simulink library "Ampere_Library"  (R2022b)
settings: Solver=FixedStepDiscrete  StartTime=0  StopTime=10.0  RelTol=1e-3  EnableMultiTasking=on
undefined symbols (not defined in the file or in its folder): A_INST_double, Dem_EventStatusType, ECU_AMBIENT_TEMPERATURE, SET_ECU_AMBIENT_TEMPERATURE, SlDemoSign, Std_ReturnType
libraries: simulink x13
(part 6 of 10)

== system Ampere_Library/Basic_Software_Operation/HW_IO/A_HWDiag ==
  note: Block with high width as the function name length depends of the name in the mask.
  note: Refer Mask Description of this Library block for detailed information.
  note: Name and data type updated through mask callback
  PhysicalSampling : FunctionCaller  FunctionPrototype=[ECU_AMBIENT_TEMPERATURE_dg,RTE_Error] = GET_DIAG_AMBIENT_TEMPERATURE()  InputArgumentSpecifications=<Enter example>  OutputArgumentSpecifications=A_INST_double(1),Std_ReturnType(1)
  ECU_AMBIENT_TEMPERATURE_dg : Outport  OutDataTypeStr=double
      settings: AttributesFormatString=DT = %<OutDataTypeStr>
  RTE_Error : Outport  Port=2  OutDataTypeStr=Enum: Std_ReturnType
      settings: AttributesFormatString=DT = %<OutDataTypeStr>
  wires:
  PhysicalSampling/1 -> ECU_AMBIENT_TEMPERATURE_dg/1
  PhysicalSampling/2 -> RTE_Error/1

== system Ampere_Library/Basic_Software_Operation/HW_IO/A_HWInput ==
  note: Block with high width as the function name length depends of the name in the mask.
  note: Name and data type updated through mask callback
  note: Refer Mask Description of this Library block for detailed information.
  PhysicalSampling : FunctionCaller  FunctionPrototype=[ECU_AMBIENT_TEMPERATURE,RTE_Error] = GET_ECU_AMBIENT_TEMPERATURE()  InputArgumentSpecifications=<Enter example>  OutputArgumentSpecifications=A_INST_double(1),Std_ReturnType(1)
  ECU_AMBIENT_TEMPERATURE : Outport  OutDataTypeStr=double
      settings: AttributesFormatString=DT = %<OutDataTypeStr>
  RTE_Error : Outport  Port=2  OutDataTypeStr=Enum: Std_ReturnType
      settings: AttributesFormatString=DT = %<OutDataTypeStr>
  wires:
  PhysicalSampling/2 -> RTE_Error/1
  PhysicalSampling/1 -> ECU_AMBIENT_TEMPERATURE/1

== system Ampere_Library/Basic_Software_Operation/HW_IO/A_HWOutput ==
  note: Name updated through mask callback
  note: Block with high width as the function name length depends of the name in the mask.
  note: Refer Mask Description of this Library block for detailed information.
  ECU_AMBIENT_TEMPERATURE : Inport
  PhysicalSampling : FunctionCaller  FunctionPrototype=SET_ECU_AMBIENT_TEMPERATURE(ECU_AMBIENT_TEMPERATURE)  InputArgumentSpecifications=A_INST_double(1)  OutputArgumentSpecifications=<Enter example>
  wires:
  ECU_AMBIENT_TEMPERATURE/1 -> PhysicalSampling/1

== system Ampere_Library/MBD_Base_Blocks/Simulink/CommonlyUsedBlocks ==
  note: Commonly used blocks
  In : Inport
  Add : Sum  InputSameDT=on  RndMeth=Zero
  Bus_Creator : BusCreator  Inputs=2
  Bus_Selector : BusSelector  OutputSignals=signal1,signal2
  Cons_val : Constant  Value=0
  Data_Type_Conversion : DataTypeConversion  SaturateOnIntegerOverflow=off
  Demux : Demux  Outputs=2
  Logical_Operator : Logic  OutDataTypeStr=boolean
  Mux : Mux  Inputs=2
  Product : Product  RndMeth=Zero
  Relational_Operator : RelationalOperator  Operator=<=  OutDataTypeStr=boolean  RndMeth=Zero
  Saturation : Saturate  RndMeth=Zero
      settings: AttributesFormatString=Max = %<UpperLimit>\nMin = %<LowerLimit>\n
  Subsystem : Subsystem
      settings: CopyFcn=set_param(gcbh,'LinkStatus','none'); set_param(gcbh,'Mask','off'); set_param(gcbh,'MaskType',''); set_param(gcbh,'MaskDescription',''); set_param(gcbh,'OpenFcn',''); set_param(gcbh,'CopyFcn','');  OpenFcn=open_system(gcbh,'force');
  Switch : Switch  Criteria=u2 ~= 0  RndMeth=Zero  SaturateOnIntegerOverflow=off
  Terminator : Terminator
  VectorConcat : Concatenate
  Out : Outport

== system Ampere_Library/MBD_Base_Blocks/Simulink/Discontinuities ==
  note: Discontinuities
  Dead_Zone : DeadZone  SaturateOnIntegerOverflow=off
      settings: AttributesFormatString=|
      | Start = %<LowerValue>
      | End = %<UpperValue>
  RateLimiter : RateLimiter  SampleTimeMode=inherited
      settings: AttributesFormatString=Init = %<InitialCondition>
  Relay : Relay
      settings: AttributesFormatString=|
      | Switch On = %<OnSwitchValue>
      | Switch Off = %<OffSwitchValue>
  Saturation : Saturate  RndMeth=Zero
      settings: AttributesFormatString=Max = %<UpperLimit>\nMin = %<LowerLimit>\n
  Saturation_Dynamic : simulink/Discontinuities/Saturation Dynamic  OutMin=[]  OutMax=[]  OutDataTypeStr=Inherit: Same as second input  OutDataType=fixdt(1, 16)  OutScaling=2^-10  RndMeth=Zero  DoSatur=off

== system Ampere_Library/MBD_Base_Blocks/Simulink/Discrete ==
  note: Discrete
  Delay : Delay  InitialCondition=0
      settings: AttributesFormatString=|
      | Init = %<InitialCondition>
      | Length = %<DelayLength>
  Discrete_State_Space : DiscreteStateSpace  SampleTime=-1
      settings: AttributesFormatString=Init = %<X0>
  TappedDelay : simulink/Discrete/Tapped Delay  vinit=0.0  samptime=-1  NumDelays=4  DelayOrder=Oldest  includeCurrent=off
      settings: AttributesFormatString=|
      | IC = %<vinit>
      | Tapped Order = %<DelayOrder>
  Unit_Delay : UnitDelay  SampleTime=-1  HasFrameUpgradeWarning=on
      settings: AttributesFormatString=Init = %<InitialCondition>

== system Ampere_Library/MBD_Base_Blocks/Simulink/Logic_and_Bit_Operations ==
  note: Logic and Bit Operations
  Bit_Clear : simulink/Logic and Bit Operations/Bit Clear  iBit=0
      settings: AttributesFormatString=ith Bit = %<iBit>
  Bit_Set : simulink/Logic and Bit Operations/Bit Set  iBit=0
      settings: AttributesFormatString=ith Bit = %<iBit>
  Bitwise_Operator : simulink/Logic and Bit Operations/Bitwise Operator  logicop=AND  UseBitMask=on  BitMask=217  BitMaskRealWorld=Stored Integer
      settings: AttributesFormatString=Bit Mask = %<BitMask>\n
  Extract_Bits : simulink/Logic and Bit Operations/Extract Bits  bitsToExtract=Range starting with most significant bit  numBits=8  bitIdxRange=[0 7]  outScalingMode=Treat bit field as an integer
      settings: AttributesFormatString=No of bits = %<numBits>
  Logical_Operator : Logic  OutDataTypeStr=boolean
  Relational_Operator : RelationalOperator  Operator=<=  OutDataTypeStr=boolean  RndMeth=Zero
  Shift_Arithmetic : ArithShift  BitShiftNumber=8

== system Ampere_Library/MBD_Base_Blocks/Simulink/Lookup_Tables ==
  note: Lookup Tables
  Direct_Lookup_Table_n_D : LookupNDDirect  DiagnosticForOutOfRangeInput=None
      settings: AttributesFormatString=Table = %<Table>
  InterpolationUsingPrelookup : Interpolation_n-D  ExtrapMethod=Clip  ValidIndexMayReachLast=on  InternalRulePriority=Speed
      settings: AttributesFormatString=Table = %<Table>
  LookupTableDynamic : simulink/Lookup Tables/Lookup Table Dynamic  LookUpMeth=Interpolation-Use End Values  OutDataType=fixdt('double')  OutScaling=[]  OutputDataTypeScalingMode=Specify via dialog  OutDataTypeStr=double  RndMeth=Zero  DoSatur=off
      settings: AttributesFormatString=DT = %<OutDataTypeStr>
  One_D_Lookup_Table : Lookup_n-D  NumberOfTableDimensions=1  BreakpointsForDimension1=[-5:5]  Table=tanh([-5:5])  ExtrapMethod=Clip  UseLastTableValue=on  InternalRulePriority=Speed  OutDataTypeStr=Inherit: Inherit from 'Table data'  RndMeth=Zero
      settings: AttributesFormatString=|
      | Table = %<Table>
      | X = %<BreakpointsForDimension1>
  Prelookup : PreLookup  BreakpointsData=[10:10:110]  UseLastBreakpoint=on  FractionDataTypeStr=fixdt(1,32,0)
      settings: AttributesFormatString=X = %<BreakpointsData>
  Two_D_Lookup_Table : Lookup_n-D  BreakpointsForDimension1=[1:3]  BreakpointsForDimension2=[1:3]  ExtrapMethod=Clip  UseLastTableValue=on  InternalRulePriority=Speed  OutDataTypeStr=Inherit: Inherit from 'Table data'  RndMeth=Zero
      settings: InputPortMap=u0,u1
      settings: AttributesFormatString=|
      | Table = %<Table>
      | X = %<BreakpointsForDimension1>
      | Y = %<BreakpointsForDimension2>

== system Ampere_Library/MBD_Base_Blocks/Simulink/Math_Operations ==
  note: Math Operations
  Abs : Abs  RndMeth=Zero  SaturateOnIntegerOverflow=off
  Add : Sum  InputSameDT=on  RndMeth=Zero
  Assignment : Assignment  IndexMode=Zero-based  IndexOptions=Index vector (dialog)  Indices=1  OutputSizes=1
      settings: AttributesFormatString=Index Mode = %<IndexMode>\n
  Divide : Product  Inputs=*/  RndMeth=Zero
  MatrixConcatenate : Concatenate  Mode=Multidimensional array  ConcatenateDimension=2
  MinMax : MinMax  InputSameDT=on  RndMeth=Zero
  Permute Dimensions : PermuteDimensions
  Product : Product  RndMeth=Zero
  Product_of_Elements : Product  Inputs=*  RndMeth=Zero
  Reshape : Reshape
  Sign : Signum
  Subtract : Sum  Inputs=+-  InputSameDT=on  RndMeth=Zero
  Sum_of_Elements : Sum  Inputs=+  InputSameDT=on  RndMeth=Zero
  VectorConcatenate : Concatenate

== system Ampere_Library/MBD_Base_Blocks/Simulink/Model_Wide_Utilities ==
  note: Model Wide Utilities
  DocBlock : simulink/Model-Wide Utilities/DocBlock  DocumentType=Text
      content=|
      | Type your documentation here
  ModelInfo : simulink/Model-Wide Utilities/Model Info  Frame=on  DisplayStringWithTags=Model Info  HorizontalTextAlignment=Center  LeftAlignmentValue=0.5

== system Ampere_Library/MBD_Base_Blocks/Simulink/Ports_and_Subsystems ==
  note: Ports & Subsystems
  In1 : Inport
  Enable : EnablePort
      settings: AttributesFormatString=%<StatesWhenEnabling>\n
  Trigger : TriggerPort  VariantControl=Variant  PortDimensions=1
  Atomic_Subsystem : Subsystem  TreatAsAtomicUnit=on
      settings: CopyFcn=set_param(gcbh,'LinkStatus','none'); set_param(gcbh,'Mask','off'); set_param(gcbh,'MaskType',''); set_param(gcbh,'MaskDescription',''); set_param(gcbh,'OpenFcn',''); set_param(gcbh,'CopyFcn','');  OpenFcn=open_system(gcbh,'force');
  CodeReuseSubsystem : Subsystem  TreatAsAtomicUnit=on
      settings: CopyFcn=set_param(gcbh,'LinkStatus','none'); set_param(gcbh,'Mask','off'); set_param(gcbh,'MaskType',''); set_param(gcbh,'MaskDescription',''); set_param(gcbh,'OpenFcn',''); set_param(gcbh,'CopyFcn','');  OpenFcn=open_system(gcbh,'force');  RTWFcnNameOpts=Use subsystem name  RTWFileNameOpts=Use function name
  Enabled_Subsystem : Subsystem  TreatAsAtomicUnit=on
      settings: CopyFcn=set_param(gcbh,'LinkStatus','none'); set_param(gcbh,'Mask','off'); set_param(gcbh,'MaskType',''); set_param(gcbh,'MaskDescription',''); set_param(gcbh,'OpenFcn',''); set_param(gcbh,'CopyFcn','');  OpenFcn=open_system(gcbh,'force');
  Enabled_and_Triggered_Subsystem : Subsystem  TreatAsAtomicUnit=on
      settings: CopyFcn=set_param(gcbh,'LinkStatus','none'); set_param(gcbh,'Mask','off'); set_param(gcbh,'MaskType',''); set_param(gcbh,'MaskDescription',''); set_param(gcbh,'OpenFcn',''); set_param(gcbh,'CopyFcn','');  OpenFcn=open_system(gcbh,'force');
  ForEachSubsystem : Subsystem  TreatAsAtomicUnit=on
      settings: CopyFcn=set_param(gcbh,'LinkStatus','breakWithoutHierarchy'); set_param(gcbh,'Mask','off'); set_param(gcbh,'MaskType',''); set_param(gcbh,'MaskDescription',''); set_param(gcbh,'OpenFcn',''); set_param(gcbh,'CopyFcn','')
  For_Iterator_Subsystem : Subsystem  TreatAsAtomicUnit=on
      settings: CopyFcn=set_param(gcbh,'LinkStatus','none'); set_param(gcbh,'Mask','off'); set_param(gcbh,'MaskType',''); set_param(gcbh,'MaskDescription',''); set_param(gcbh,'OpenFcn',''); set_param(gcbh,'CopyFcn','');  OpenFcn=open_system(gcbh,'force');
  Function_Call_Subsystem : Subsystem  TreatAsAtomicUnit=on
      settings: CopyFcn=set_param(gcbh,'LinkStatus','none'); set_param(gcbh,'Mask','off'); set_param(gcbh,'MaskType',''); set_param(gcbh,'MaskDescription',''); set_param(gcbh,'OpenFcn',''); set_param(gcbh,'CopyFcn','');  OpenFcn=open_system(gcbh,'force');
  If : If
  If_Action_Subsystem : Subsystem  TreatAsAtomicUnit=on
      settings: CopyFcn=set_param(gcbh,'LinkStatus','none'); set_param(gcbh,'Mask','off'); set_param(gcbh,'MaskType',''); set_param(gcbh,'MaskDescription',''); set_param(gcbh,'OpenFcn',''); set_param(gcbh,'CopyFcn','');  OpenFcn=open_system(gcbh,'force');
  Model : ModelReference  SimulationMode=Normal
  Model_Variants : Subsystem  Variant=on
      settings: AttributesFormatString=Active variants=%<ActiveVariant>\n
  Subsystem : Subsystem
      settings: CopyFcn=set_param(gcbh,'LinkStatus','none'); set_param(gcbh,'Mask','off'); set_param(gcbh,'MaskType',''); set_param(gcbh,'MaskDescription',''); set_param(gcbh,'OpenFcn',''); set_param(gcbh,'CopyFcn','');  OpenFcn=open_system(gcbh,'force');
  Switch_Case : SwitchCase
  Switch_Case_Action_Subsystem : Subsystem  TreatAsAtomicUnit=on
      settings: CopyFcn=set_param(gcbh,'LinkStatus','none'); set_param(gcbh,'Mask','off'); set_param(gcbh,'MaskType',''); set_param(gcbh,'MaskDescription',''); set_param(gcbh,'OpenFcn',''); set_param(gcbh,'CopyFcn','');  OpenFcn=open_system(gcbh,'force');
  Triggered_Subsystem : Subsystem  TreatAsAtomicUnit=on
      settings: CopyFcn=set_param(gcbh,'LinkStatus','none'); set_param(gcbh,'Mask','off'); set_param(gcbh,'MaskType',''); set_param(gcbh,'MaskDescription',''); set_param(gcbh,'OpenFcn',''); set_param(gcbh,'CopyFcn','');  OpenFcn=open_system(gcbh,'force');
  Variant_subsystem : Subsystem  Variant=on
      settings: AttributesFormatString=Active variants=%<ActiveVariant>\n  CopyFcn=set_param(gcbh,'LinkStatus','none'); set_param(gcbh,'Mask','off'); set_param(gcbh,'MaskType',''); set_param(gcbh,'MaskDescription',''); set_param(gcbh,'OpenFcn',''); set_param(gcbh,'CopyFcn','');
  While_Iterator_Subsystem : Subsystem  TreatAsAtomicUnit=on
      settings: CopyFcn=set_param(gcbh,'LinkStatus','none'); set_param(gcbh,'Mask','off'); set_param(gcbh,'MaskType',''); set_param(gcbh,'MaskDescription',''); set_param(gcbh,'OpenFcn',''); set_param(gcbh,'CopyFcn','');  OpenFcn=open_system(gcbh,'force');
  Out1 : Outport

== system Ampere_Library/MBD_Base_Blocks/Simulink/Signal_Attributes ==
  note: Signal Attributes
  BustoVector : BusToVector
  DataTypeDuplicate : DataTypeDuplicate
  Data_Type_Conversion : DataTypeConversion  SaturateOnIntegerOverflow=off
  SignalConversion : SignalConversion  OverrideOpt=off

== system Ampere_Library/MBD_Base_Blocks/Simulink/Signal_Routing ==
  note: Signal Routing
  BusAssignment : BusAssignment  AssignedSignals=signal1
  Bus_Creator : BusCreator  Inputs=2
      settings: CopyFcn=set_param(gcbh,'ShowName','off','CopyFcn','')
  Bus_Selector : BusSelector  OutputSignals=signal1,signal2
      settings: CopyFcn=set_param(gcbh,'ShowName','off','CopyFcn','')
  Demux : Demux  Outputs=2
      settings: CopyFcn=set_param(gcbh,'ShowName','off','CopyFcn','')
  From : From
  Goto : Goto
  IndexVector : MultiPortSwitch  DataPortOrder=Zero-based contiguous  Inputs=1  zeroidx=on  RndMeth=Zero  SaturateOnIntegerOverflow=off
  Merge : Merge
      settings: AttributesFormatString=Init = %<InitialOutput>
  Multiport_Switch : MultiPortSwitch  DataPortOrder=Zero-based contiguous  DataPortForDefault=Additional data port  DiagnosticForDefault=None  zeroidx=on  RndMeth=Zero  SaturateOnIntegerOverflow=off
  Mux : Mux  Inputs=2
      settings: CopyFcn=set_param(gcbh,'ShowName','off','CopyFcn','')
  Selector : Selector  IndexMode=Zero-based  IndexOptions=Index vector (port)  Indices=[1 3]  OutputSizes=1
  Switch : Switch  Criteria=u2 ~= 0  RndMeth=Zero  SaturateOnIntegerOverflow=off

== system Ampere_Library/MBD_Base_Blocks/Simulink/Sinks ==
  note: Sinks
  Terminator : Terminator
  Out : Outport

== system Ampere_Library/MBD_Base_Blocks/Simulink/Sources ==
  note: Sources
  In : Inport
  Constant : Constant  Value=0
  EnumeratedConstant : simulink/Sources/Enumerated Constant  OutDataTypeStr=Enum: SlDemoSign  Value=SlDemoSign.Positive  SampleTime=inf
      settings: AttributesFormatString=Enum
  Ground : Ground

== system Ampere_Library/MBD_Base_Blocks/Simulink/User_Defined_Functions ==
  note: User_Defined_Functions
  FunctionCaller : FunctionCaller  FunctionPrototype=y = f(u)  InputArgumentSpecifications=<Enter example>  OutputArgumentSpecifications=<Enter example>
  Initialize_Function : Subsystem  TreatAsAtomicUnit=on
  MATLAB_Function : MATLAB Function  TreatAsAtomicUnit=on
  Simulink_Function : Subsystem  TreatAsAtomicUnit=on
      settings: CopyFcn=set_param(gcbh,'LinkStatus','breakWithoutHierarchy'); set_param(gcbh,'Mask','off'); set_param(gcbh,'MaskType',''); set_param(gcbh,'MaskDescription',''); set_param(gcbh,'OpenFcn',''); set_param(gcbh,'CopyFcn','')

== system Ampere_Library/User_Defined_Libraries/Discontinuities/A_DetectSaturation ==
  note: Refer Mask Description of this Library block for detailed information.
  Upper : Inport
  In : Inport  Port=2
  Lower : Inport  Port=3
  LogicalOperator : Logic  OutDataTypeStr=boolean
  LogicalOperator1 : Logic  Operator=NOT  OutDataTypeStr=boolean
  LogicalOperator2 : Logic  Operator=NOT  OutDataTypeStr=boolean
  Max : MinMax  Function=max  Inputs=2  InputSameDT=on  RndMeth=Zero
      settings: AttributesFormatString=SAT = %<SaturateOnIntegerOverflow>
  Min : MinMax  Inputs=2  InputSameDT=on  RndMeth=Zero
      settings: AttributesFormatString=SAT = %<SaturateOnIntegerOverflow>
  RelationalOperator2 : RelationalOperator  Operator=>  OutDataTypeStr=boolean  RndMeth=Zero
  RelationalOperator3 : RelationalOperator  Operator=<  OutDataTypeStr=boolean  RndMeth=Zero
  RelationalOperator4 : RelationalOperator  Operator=<=  OutDataTypeStr=boolean  RndMeth=Zero
  RelationalOperator5 : RelationalOperator  OutDataTypeStr=boolean  RndMeth=Zero
  SATMAX : Constant  Value=SatMax
  SATMAX1 : Constant  Value=SatMax
  SATMIN : Constant  Value=Satmin
  SATPAS : Constant  Value=SatPas
  Switch{1..4} (4 alike) : Switch  Criteria=u2 ~= 0  RndMeth=Zero  SaturateOnIntegerOverflow=off
  UP_EQ_LOW : Constant  Value=UpEqLow
  Out : Outport
  sat : Outport  Port=2
  wires:
  Lower/1 -> Max/2, [Lower]
  Min/1 -> Out/1, RelationalOperator4/1, RelationalOperator5/1
  [Lower] -> RelationalOperator4/2
  Max/1 -> Min/1
  [Upper] -> RelationalOperator5/2
  LogicalOperator2/1 -> LogicalOperator/1
  Upper/1 -> [Upper], Min/2
  SATPAS/1 -> Switch4/3
  Switch1/1 -> Switch3/3
  [Upper] -> RelationalOperator2/1, RelationalOperator3/1
  RelationalOperator2/1 -> LogicalOperator2/1
  SATMAX1/1 -> Switch3/1
  Switch2/1 -> sat/1
  RelationalOperator4/1 -> Switch4/2
  RelationalOperator3/1 -> LogicalOperator1/1, Switch3/2
  RelationalOperator5/1 -> Switch1/2
  Switch3/1 -> Switch2/3
  SATMAX/1 -> Switch1/1
  [Lower] -> RelationalOperator2/2, RelationalOperator3/2
  In/1 -> Max/1
  LogicalOperator1/1 -> LogicalOperator/2
  LogicalOperator/1 -> Switch2/2
  UP_EQ_LOW/1 -> Switch2/1
  Switch4/1 -> Switch1/3
  SATMIN/1 -> Switch4/1

== system Ampere_Library/User_Defined_Libraries/Discontinuities/A_HiThresHys_HighIncl ==
  note: Refer Mask Description of this Library block for detailed information.
  note: hflg = OFF
  note: hflg = ON
  val : Inport
  thrs : Inport  Port=2
  hysw : Inport  Port=3
  NOT : Logic  Operator=NOT  Inputs=1  OutDataTypeStr=boolean
  RelOperator1 : RelationalOperator  Operator=>  OutDataTypeStr=boolean  RndMeth=Zero
  RelOperator2 : RelationalOperator  Operator=<  OutDataTypeStr=boolean  RndMeth=Zero
  Sum : Sum  InputSameDT=on  RndMeth=Zero
      settings: AttributesFormatString=SAT = %<SaturateOnIntegerOverflow>
  Switch : Switch  Criteria=u2 ~= 0  RndMeth=Zero  SaturateOnIntegerOverflow=off
  Unit_Delay : UnitDelay  InitialCondition=Initial_condition  SampleTime=-1  HasFrameUpgradeWarning=on
      settings: AttributesFormatString=Init = %<InitialCondition>\n
  flag : Outport
  wires:
  NOT/1 -> flag/1, Unit_Delay/1
  Unit_Delay/1 -> Switch/2
  RelOperator2/1 -> Switch/3
  RelOperator1/1 -> Switch/1
  hysw/1 -> Sum/2
  Switch/1 -> NOT/1
  Sum/1 -> RelOperator1/2
  thrs/1 -> RelOperator1/1, RelOperator2/2
  val/1 -> RelOperator2/1, Sum/1

== system Ampere_Library/User_Defined_Libraries/Discontinuities/A_HiThresHys_LowIncl ==
  note: Refer Mask Description of this Library block for detailed information.
  note: hflg = OFF
  note: hflg = ON
  val : Inport
  thrs : Inport  Port=2
  hysw : Inport  Port=3
  NOT : Logic  Operator=NOT  Inputs=1  OutDataTypeStr=boolean
  RelationOperator1 : RelationalOperator  Operator=<=  OutDataTypeStr=boolean  RndMeth=Zero
  RelationalOperator : RelationalOperator  OutDataTypeStr=boolean  RndMeth=Zero
  Sum : Sum  InputSameDT=on  RndMeth=Zero
      settings: AttributesFormatString=SAT = %<SaturateOnIntegerOverflow>
  Switch : Switch  Criteria=u2 ~= 0  RndMeth=Zero  SaturateOnIntegerOverflow=off
  Unit_Delay : UnitDelay  InitialCondition=Initial_condition  SampleTime=-1  HasFrameUpgradeWarning=on
      settings: AttributesFormatString=Init = %<InitialCondition>\n
  flag : Outport
  wires:
  NOT/1 -> flag/1, Unit_Delay/1
  Unit_Delay/1 -> Switch/2
  RelationOperator1/1 -> Switch/3
  RelationalOperator/1 -> Switch/1
  hysw/1 -> Sum/2
  Switch/1 -> NOT/1
  Sum/1 -> RelationalOperator/2
  val/1 -> RelationOperator1/1, Sum/1
  thrs/1 -> RelationalOperator/1, RelationOperator1/2

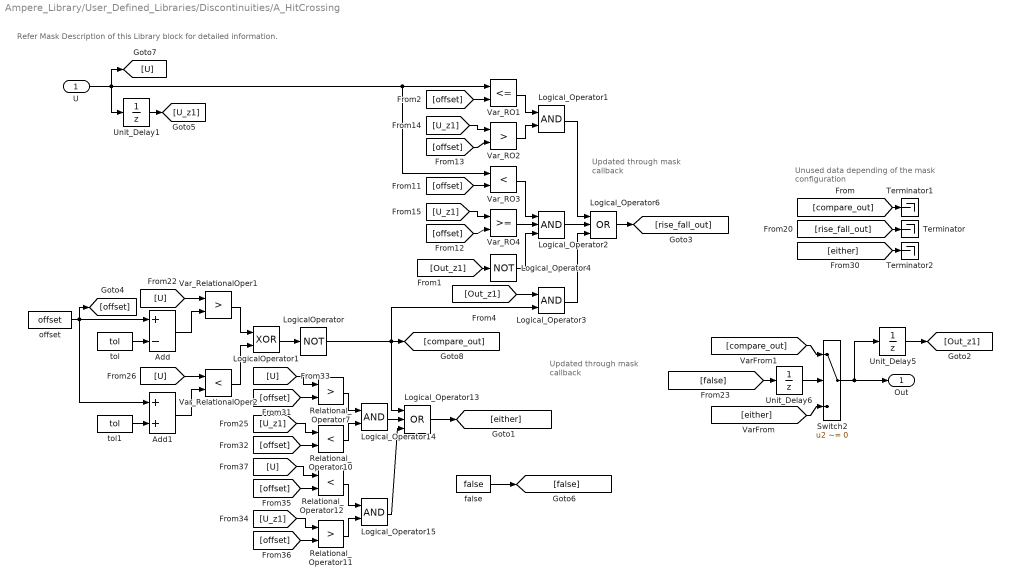
== system Ampere_Library/User_Defined_Libraries/Discontinuities/A_HitCrossing ==
  note: Updated through
      | mask callback
  note: Refer Mask Description of this Library block for detailed information.
  note: Unused data depending
      | of the mask configuration
  note: Updated through
      | mask callback
  U : Inport
  Add : Sum  Inputs=+-  InputSameDT=on  RndMeth=Zero
      settings: AttributesFormatString=SAT = %<SaturateOnIntegerOverflow>
  Add1 : Sum  InputSameDT=on  RndMeth=Zero
      settings: AttributesFormatString=SAT = %<SaturateOnIntegerOverflow>
  LogicalOperator : Logic  Operator=NOT  OutDataTypeStr=boolean
  LogicalOperator1 : Logic  Operator=XOR  OutDataTypeStr=boolean
  Logical_Operator{1,3,14..15} (4 alike) : Logic  OutDataTypeStr=boolean
  Logical_Operator13 : Logic  Operator=OR  Inputs=3  OutDataTypeStr=boolean
  Logical_Operator2 : Logic  Inputs=3  OutDataTypeStr=boolean
  Logical_Operator4 : Logic  Operator=NOT  OutDataTypeStr=boolean
  Logical_Operator6 : Logic  Operator=OR  Inputs=3  OutDataTypeStr=boolean
  Relational_Operator10 : RelationalOperator  Operator=<  OutDataTypeStr=boolean  RndMeth=Zero
  Relational_Operator11 : RelationalOperator  Operator=>  OutDataTypeStr=boolean  RndMeth=Zero
  Relational_Operator12 : RelationalOperator  Operator=<  OutDataTypeStr=boolean  RndMeth=Zero
  Relational_Operator7 : RelationalOperator  Operator=>  OutDataTypeStr=boolean  RndMeth=Zero
  Switch2 : Switch  Criteria=u2 ~= 0  RndMeth=Zero  SaturateOnIntegerOverflow=off
  Terminator : Terminator
  Terminator1 : Terminator
  Terminator2 : Terminator
  Unit_Delay1 : UnitDelay  InitialCondition=INI_VAL  SampleTime=-1  HasFrameUpgradeWarning=on
      settings: AttributesFormatString=Init = %<InitialCondition>
  Unit_Delay5 : UnitDelay  InitialCondition=false  SampleTime=-1  HasFrameUpgradeWarning=on
      settings: AttributesFormatString=Init = %<InitialCondition>
  Unit_Delay6 : UnitDelay  InitialCondition=true  SampleTime=-1  HasFrameUpgradeWarning=on
      settings: AttributesFormatString=Init = %<InitialCondition>
  Var_RO1 : RelationalOperator  Operator=<=  OutDataTypeStr=boolean  RndMeth=Zero
  Var_RO2 : RelationalOperator  Operator=>  OutDataTypeStr=boolean  RndMeth=Zero
  Var_RO3 : RelationalOperator  Operator=<  OutDataTypeStr=boolean  RndMeth=Zero
  Var_RO4 : RelationalOperator  OutDataTypeStr=boolean  RndMeth=Zero
  Var_RelationalOper1 : RelationalOperator  Operator=>  OutDataTypeStr=boolean  RndMeth=Zero
  Var_RelationalOper2 : RelationalOperator  Operator=<  OutDataTypeStr=boolean  RndMeth=Zero
  false : Constant  Value=false
  offset : Constant  Value=offset  OutDataTypeStr=Inherit: Inherit via back propagation
  tol : Constant  Value=tol  OutDataTypeStr=Inherit: Inherit via back propagation
  tol1 : Constant  Value=tol  OutDataTypeStr=Inherit: Inherit via back propagation
  Out : Outport
  wires:
  [offset] -> Relational_Operator7/2
  Var_RO1/1 -> Logical_Operator1/1
  Logical_Operator6/1 -> [rise_fall_out]
  Unit_Delay5/1 -> [Out_z1]
  Var_RelationalOper2/1 -> LogicalOperator1/2
  LogicalOperator1/1 -> LogicalOperator/1
  Var_RO2/1 -> Logical_Operator1/2
  Add1/1 -> Var_RelationalOper2/2
  Unit_Delay1/1 -> [U_z1]
  [false] -> Unit_Delay6/1
  [compare_out] -> Switch2/1
  [offset] -> Relational_Operator10/2
  Logical_Operator13/1 -> [either]
  [U_z1] -> Relational_Operator10/1
  [offset] -> Relational_Operator12/2
  Relational_Operator11/1 -> Logical_Operator15/2
  Logical_Operator15/1 -> Logical_Operator13/3
  [U_z1] -> Relational_Operator11/1
  Relational_Operator7/1 -> Logical_Operator14/1
  Relational_Operator10/1 -> Logical_Operator14/2
  [offset] -> Var_RO3/2
  Unit_Delay6/1 -> Switch2/2
  Logical_Operator2/1 -> Logical_Operator6/2
  [U_z1] -> Var_RO4/1
  Logical_Operator1/1 -> Logical_Operator6/1
  [Out_z1] -> Logical_Operator4/1
  [offset] -> Relational_Operator11/2
  [U] -> Var_RelationalOper2/1
  U/1 -> Var_RO1/1, Var_RO3/1, [U], Unit_Delay1/1
  [offset] -> Var_RO1/2
  [U] -> Relational_Operator12/1
  Var_RO3/1 -> Logical_Operator2/1
  Switch2/1 -> Out/1, Unit_Delay5/1
  Relational_Operator12/1 -> Logical_Operator15/1
  [U] -> Relational_Operator7/1
  [offset] -> Var_RO4/2
  [either] -> Switch2/3
  Logical_Operator14/1 -> Logical_Operator13/2
  offset/1 -> Add/1, [offset], Add1/1
  [either] -> Terminator2/1
  tol1/1 -> Add1/2
  [U] -> Var_RelationalOper1/1
  [rise_fall_out] -> Terminator/1
  [Out_z1] -> Logical_Operator3/1
  [offset] -> Var_RO2/2
  tol/1 -> Add/2
  Logical_Operator3/1 -> Logical_Operator6/3
  Logical_Operator4/1 -> Logical_Operator2/3
  Add/1 -> Var_RelationalOper1/2
  Var_RelationalOper1/1 -> LogicalOperator1/1
  [U_z1] -> Var_RO2/1
  Var_RO4/1 -> Logical_Operator2/2
  false/1 -> [false]
  LogicalOperator/1 -> Logical_Operator3/2, Logical_Operator13/1, [compare_out]
  [compare_out] -> Terminator1/1

== system Ampere_Library/User_Defined_Libraries/Discontinuities/A_Hysteresis ==
  note: Refer Mask Description of this Library block for detailed information.
  High : Inport
  In : Inport  Port=2
  Low : Inport  Port=3
  FixPt_Relational_Operator : RelationalOperator  OutDataTypeStr=boolean  ZeroCross=off  RndMeth=Zero
  FixPt_Relational_Operator1 : RelationalOperator  Operator=<=  OutDataTypeStr=boolean  ZeroCross=off  RndMeth=Zero
  Logical_Operator : Logic  Operator=OR  OutDataTypeStr=boolean
  Logical_Operator1 : Logic  Operator=NOT  OutDataTypeStr=boolean
  Logical_Operator2 : Logic  OutDataTypeStr=boolean
  Unit_Delay : UnitDelay  InitialCondition=HysIni  SampleTime=-1  HasFrameUpgradeWarning=on
      settings: AttributesFormatString=Init = %<InitialCondition>
  Out : Outport
  wires:
  Logical_Operator/1 -> Logical_Operator2/1
  Logical_Operator1/1 -> Logical_Operator2/2
  Unit_Delay/1 -> Logical_Operator/1
  High/1 -> FixPt_Relational_Operator/2
  Low/1 -> FixPt_Relational_Operator1/2
  FixPt_Relational_Operator/1 -> Logical_Operator/2
  FixPt_Relational_Operator1/1 -> Logical_Operator1/1
  In/1 -> FixPt_Relational_Operator1/1, FixPt_Relational_Operator/1
  Logical_Operator2/1 -> Out/1, Unit_Delay/1

== system Ampere_Library/User_Defined_Libraries/Discontinuities/A_Hysteresis_Ext_Values ==
  note: Updated through
      | mask callback
  note: A_UnitDelayExternalIC
  note: Refer Mask Description of this Library block for detailed information.
  Inp : Inport
  Threshold1 : Inport  Port=2
  Threshold2 : Inport  Port=3
  Value1 : Inport  Port=4
  Value2 : Inport  Port=5
  DefaultValue : Inport  Port=6
  FixPtUnitDelay2 : UnitDelay  DisableCoverage=on  InitialCondition=false  SampleTime=-1  HasFrameUpgradeWarning=on
      settings: AttributesFormatString=Init = %<InitialCondition>
  FixPt_Unit_Delay1 : UnitDelay  DisableCoverage=on  InitialCondition=UDEIC_zero  SampleTime=-1  HasFrameUpgradeWarning=on
      settings: AttributesFormatString=Init = %<InitialCondition>
  RO_Th1Strict : RelationalOperator  OutDataTypeStr=boolean  RndMeth=Zero
  RO_Th2Strict : RelationalOperator  OutDataTypeStr=boolean  RndMeth=Zero
  Switch : Switch  Criteria=u2 ~= 0  RndMeth=Zero  SaturateOnIntegerOverflow=off
      settings: AttributesFormatString=SAT = %<SaturateOnIntegerOverflow>
  Switch1 : Switch  Criteria=u2 ~= 0  RndMeth=Zero  SaturateOnIntegerOverflow=off
      settings: AttributesFormatString=SAT = %<SaturateOnIntegerOverflow>
  SwitchInit : Switch  Criteria=u2 ~= 0  RndMeth=Zero  ZeroCross=off  SaturateOnIntegerOverflow=off
      settings: AttributesFormatString=SAT = %<SaturateOnIntegerOverflow>
  true : Constant  DisableCoverage=on  Value=true
  Out : Outport
  wires:
  SwitchInit/1 -> Switch/3
  Switch/1 -> Switch1/3
  RO_Th2Strict/1 -> Switch/2
  RO_Th1Strict/1 -> Switch1/2
  Threshold1/1 -> RO_Th1Strict/1
  Threshold2/1 -> RO_Th2Strict/2
  Inp/1 -> RO_Th1Strict/2, RO_Th2Strict/1
  DefaultValue/1 -> SwitchInit/3
  Switch1/1 -> Out/1, FixPt_Unit_Delay1/1
  true/1 -> FixPtUnitDelay2/1
  FixPtUnitDelay2/1 -> SwitchInit/2
  FixPt_Unit_Delay1/1 -> SwitchInit/1
  Value2/1 -> Switch/1
  Value1/1 -> Switch1/1

== system Ampere_Library/User_Defined_Libraries/Discontinuities/A_Hysteresis_WithConf ==
  note: A_UnitDelayExternalIC
  note: Updated through
      | mask callback
  note: Refer Mask Description of this Library block for detailed information.
  Inp : Inport
  Threshold1 : Inport  Port=2
  Threshold2 : Inport  Port=3
  Value1 : Inport  Port=4
  Value2 : Inport  Port=5
  DefaultValue : Inport  Port=6
  Timestep : Inport  Port=7
  ConfirmationTime : Inport  Port=8
  Demux : Demux  Outputs=2
  FixPtUnitDelay2 : UnitDelay  DisableCoverage=on  InitialCondition=false  SampleTime=-1  HasFrameUpgradeWarning=on
      settings: AttributesFormatString=Init = %<InitialCondition>
  FixPt_Unit_Delay1 : UnitDelay  DisableCoverage=on  InitialCondition=UDEIC_zero  SampleTime=-1  HasFrameUpgradeWarning=on
      settings: AttributesFormatString=Init = %<InitialCondition>
  ForEachTurnOnDelay : Subsystem  TreatAsAtomicUnit=on
      settings: RTWSystemCode=Inline
  Init : Switch  Criteria=u2 ~= 0  RndMeth=Zero  ZeroCross=off  SaturateOnIntegerOverflow=off
      settings: AttributesFormatString=SAT = %<SaturateOnIntegerOverflow>
  Mux : Mux  Inputs=2
  RO_Th1Strict : RelationalOperator  OutDataTypeStr=boolean  RndMeth=Zero
  RO_Th2Strict : RelationalOperator  Operator=>  OutDataTypeStr=boolean  RndMeth=Zero
  Switch : Switch  Criteria=u2 ~= 0  RndMeth=Zero  SaturateOnIntegerOverflow=off
      settings: AttributesFormatString=SAT = %<SaturateOnIntegerOverflow>
  Switch1 : Switch  Criteria=u2 ~= 0  RndMeth=Zero  SaturateOnIntegerOverflow=off
      settings: AttributesFormatString=SAT = %<SaturateOnIntegerOverflow>
  true : Constant  DisableCoverage=on  Value=true
  Out : Outport
  wires:
  Threshold1/1 -> RO_Th1Strict/1
  Timestep/1 -> ForEachTurnOnDelay/3(Timestep)
  Value1/1 -> Switch1/1
  Demux/2 -> Switch/2
  Value2/1 -> Switch/1
  Init/1 -> Switch/3
  Demux/1 -> Switch1/2
  Inp/1 -> RO_Th2Strict/1, RO_Th1Strict/2
  Switch/1 -> Switch1/3
  Threshold2/1 -> RO_Th2Strict/2
  RO_Th1Strict/1 -> Mux/1
  RO_Th2Strict/1 -> Mux/2
  Mux/1 -> ForEachTurnOnDelay/2(Signal)  "Signal"
  ConfirmationTime/1 -> ForEachTurnOnDelay/1(ConfirmationTime)
  ForEachTurnOnDelay/1(Outx) -> Demux/1
  DefaultValue/1 -> Init/3
  FixPt_Unit_Delay1/1 -> Init/1
  FixPtUnitDelay2/1 -> Init/2
  true/1 -> FixPtUnitDelay2/1
  Switch1/1 -> Out/1, FixPt_Unit_Delay1/1

== system Ampere_Library/User_Defined_Libraries/Discontinuities/A_LowThresHys_HighIncl ==
  note: Refer Mask Description of this Library block for detailed information.
  val : Inport
  thrs : Inport  Port=2
  hysw : Inport  Port=3
  NOT : Logic  Operator=NOT  Inputs=1  OutDataTypeStr=boolean
  Sum : Sum  Inputs=+-  InputSameDT=on  RndMeth=Zero
      settings: AttributesFormatString=SAT = %<SaturateOnIntegerOverflow>
  Switch : Switch  Criteria=u2 ~= 0  RndMeth=Zero  SaturateOnIntegerOverflow=off
      settings: AttributesFormatString=SAT = %<SaturateOnIntegerOverflow>
  UnitDelay : UnitDelay  InitialCondition=Init_Val  SampleTime=-1  HasFrameUpgradeWarning=on
      settings: AttributesFormatString=Init = %<InitialCondition>\n
  hflg_OFF : RelationalOperator  Operator=<=  OutDataTypeStr=boolean  RndMeth=Zero
  hflg_ON : RelationalOperator  OutDataTypeStr=boolean  RndMeth=Zero
  flag : Outport
  wires:
  thrs/1 -> hflg_ON/2, hflg_OFF/1
  val/1 -> hflg_ON/1, Sum/1
  hflg_ON/1 -> Switch/3
  hflg_OFF/1 -> Switch/1
  Sum/1 -> hflg_OFF/2
  hysw/1 -> Sum/2
  NOT/1 -> Switch/2
  UnitDelay/1 -> NOT/1
  Switch/1 -> UnitDelay/1, flag/1

== system Ampere_Library/User_Defined_Libraries/Discontinuities/A_LowThresHys_LowIncl ==
  note: Refer Mask Description of this Library block for detailed information.
  val : Inport
  thrs : Inport  Port=2
  hysw : Inport  Port=3
  NOT : Logic  Operator=NOT  Inputs=1  OutDataTypeStr=boolean
  Sum : Sum  Inputs=+-  InputSameDT=on  RndMeth=Zero
      settings: AttributesFormatString=SAT = %<SaturateOnIntegerOverflow>
  Switch : Switch  Criteria=u2 ~= 0  RndMeth=Zero  SaturateOnIntegerOverflow=off
      settings: AttributesFormatString=SAT = %<SaturateOnIntegerOverflow>
  UnitDelay : UnitDelay  InitialCondition=flag_init  SampleTime=-1  HasFrameUpgradeWarning=on
      settings: AttributesFormatString=Init = %<InitialCondition>\n
  hflg_OFF : RelationalOperator  Operator=<  OutDataTypeStr=boolean  RndMeth=Zero
  hflg_ON : RelationalOperator  Operator=>  OutDataTypeStr=boolean  RndMeth=Zero
  flag : Outport
  wires:
  UnitDelay/1 -> NOT/1
  Switch/1 -> UnitDelay/1, flag/1
  hflg_ON/1 -> Switch/3
  hflg_OFF/1 -> Switch/1
  hysw/1 -> Sum/2
  NOT/1 -> Switch/2
  Sum/1 -> hflg_OFF/2
  thrs/1 -> hflg_OFF/1, hflg_ON/2
  val/1 -> Sum/1, hflg_ON/1

== system Ampere_Library/User_Defined_Libraries/Discontinuities/A_MaxSaturation ==
  note: Refer Mask Description of this Library block for detailed information.
  u : Inport
  Max : Constant  Value=Max  OutDataTypeStr=Inherit: Inherit via back propagation  LockScale=on
  MinMax : MinMax  Inputs=2  InputSameDT=on  RndMeth=Zero
      settings: AttributesFormatString=SAT = %<SaturateOnIntegerOverflow>
  y : Outport
  wires:
  Max/1 -> MinMax/2
  MinMax/1 -> y/1
  u/1 -> MinMax/1

== system Ampere_Library/User_Defined_Libraries/Discontinuities/A_MinSaturation ==
  note: Refer Mask Description of this Library block for detailed information.
  u : Inport
  Min : Constant  Value=Min  OutDataTypeStr=Inherit: Inherit via back propagation
  MinMax : MinMax  Function=max  Inputs=2  InputSameDT=on  RndMeth=Zero
      settings: AttributesFormatString=SAT = %<SaturateOnIntegerOverflow>
  y : Outport
  wires:
  MinMax/1 -> y/1
  u/1 -> MinMax/1
  Min/1 -> MinMax/2

== system Ampere_Library/User_Defined_Libraries/Discontinuities/A_NegativeDecreaseDeadZone ==
  note: Refer Mask Description of this Library block for detailed information.
  New_value : Inport
  DeadBand : Constant  Value=DeadBand  OutDataTypeStr=Inherit: Inherit via back propagation
  INIVAL : Constant  Value=IniVal  OutDataTypeStr=Inherit: Inherit via back propagation
  MinMax : MinMax  Inputs=2  InputSameDT=on  RndMeth=Zero
      settings: AttributesFormatString=SAT = %<SaturateOnIntegerOverflow>
  Operateur_Logicals : Logic  Operator=OR  OutDataTypeStr=boolean
  Relational_Operator : RelationalOperator  OutDataTypeStr=boolean  RndMeth=Zero
  Relational_Operator1 : RelationalOperator  Operator=<=  OutDataTypeStr=boolean  RndMeth=Zero
  Sum : Sum  Inputs=+-  InputSameDT=on  RndMeth=Zero
      settings: AttributesFormatString=SAT = %<SaturateOnIntegerOverflow>
  Switch : Switch  Criteria=u2 ~= 0  RndMeth=Zero  SaturateOnIntegerOverflow=off
      settings: AttributesFormatString=SAT = %<SaturateOnIntegerOverflow>
  Unit_Delay : UnitDelay  InitialCondition=IniVal  SampleTime=-1  HasFrameUpgradeWarning=on
      settings: AttributesFormatString=Init = %<InitialCondition>
  Freezed_value : Outport
  wires:
  Switch/1 -> Freezed_value/1, Unit_Delay/1
  Sum/1 -> Relational_Operator1/2
  Relational_Operator1/1 -> Operateur_Logicals/1
  Operateur_Logicals/1 -> Switch/2
  Relational_Operator/1 -> Operateur_Logicals/2
  New_value/1 -> MinMax/1
  INIVAL/1 -> MinMax/2
  MinMax/1 -> Relational_Operator1/1, Relational_Operator/1, Switch/1
  DeadBand/1 -> Sum/2
  Unit_Delay/1 -> Sum/1, Relational_Operator/2, Switch/3

== system Ampere_Library/User_Defined_Libraries/Discontinuities/A_PositiveIncreaseDeadZone ==
  note: Refer Mask Description of this Library block for detailed information.
  New_value : Inport
  DeadBand : Constant  Value=DeadBand  OutDataTypeStr=Inherit: Inherit via back propagation
  INIVAL : Constant  Value=IniVal  OutDataTypeStr=Inherit: Inherit via back propagation
  Init_0 : UnitDelay  InitialCondition=IniVal  SampleTime=-1  HasFrameUpgradeWarning=on
      settings: AttributesFormatString=Init = %<InitialCondition>
  MinMax : MinMax  Function=max  Inputs=2  InputSameDT=on  RndMeth=Zero
      settings: AttributesFormatString=SAT = %<SaturateOnIntegerOverflow>
  Operateur_Logicals : Logic  Operator=OR  OutDataTypeStr=boolean
  Relational_Operator : RelationalOperator  Operator=<=  OutDataTypeStr=boolean  RndMeth=Zero
  Relational_Operator1 : RelationalOperator  OutDataTypeStr=boolean  RndMeth=Zero
  Sum : Sum  InputSameDT=on  RndMeth=Zero
      settings: AttributesFormatString=SAT = %<SaturateOnIntegerOverflow>
  Switch : Switch  Criteria=u2 ~= 0  RndMeth=Zero  SaturateOnIntegerOverflow=off
      settings: AttributesFormatString=SAT = %<SaturateOnIntegerOverflow>
  Freezed_value : Outport
  wires:
  Switch/1 -> Init_0/1, Freezed_value/1
  Sum/1 -> Relational_Operator1/2
  Relational_Operator1/1 -> Operateur_Logicals/1
  Init_0/1 -> Sum/2, Relational_Operator/2, Switch/3
  Operateur_Logicals/1 -> Switch/2
  Relational_Operator/1 -> Operateur_Logicals/2
  MinMax/1 -> Relational_Operator/1, Relational_Operator1/1, Switch/1
  New_value/1 -> MinMax/1
  INIVAL/1 -> MinMax/2
  DeadBand/1 -> Sum/1

== system Ampere_Library/User_Defined_Libraries/Discontinuities/A_Relay ==
  note: Refer Mask Description of this Library block for detailed information.
  In : Inport
  High : Inport  Port=2
  Low : Inport  Port=3
  RelationalOperator1 : RelationalOperator  OutDataTypeStr=boolean  RndMeth=Zero
  RelationalOperator2 : RelationalOperator  OutDataTypeStr=boolean  RndMeth=Zero
  Switch : Switch  Criteria=u2 ~= 0  RndMeth=Zero  SaturateOnIntegerOverflow=off
  UnitDelay : UnitDelay  InitialCondition=false  SampleTime=-1  HasFrameUpgradeWarning=on
      settings: AttributesFormatString=Init = %<InitialCondition>
  Out : Outport
  wires:
  High/1 -> RelationalOperator2/2
  UnitDelay/1 -> Switch/2
  RelationalOperator1/1 -> Switch/1
  RelationalOperator2/1 -> Switch/3
  In/1 -> RelationalOperator1/1, RelationalOperator2/1
  Low/1 -> RelationalOperator1/2
  Switch/1 -> Out/1, UnitDelay/1

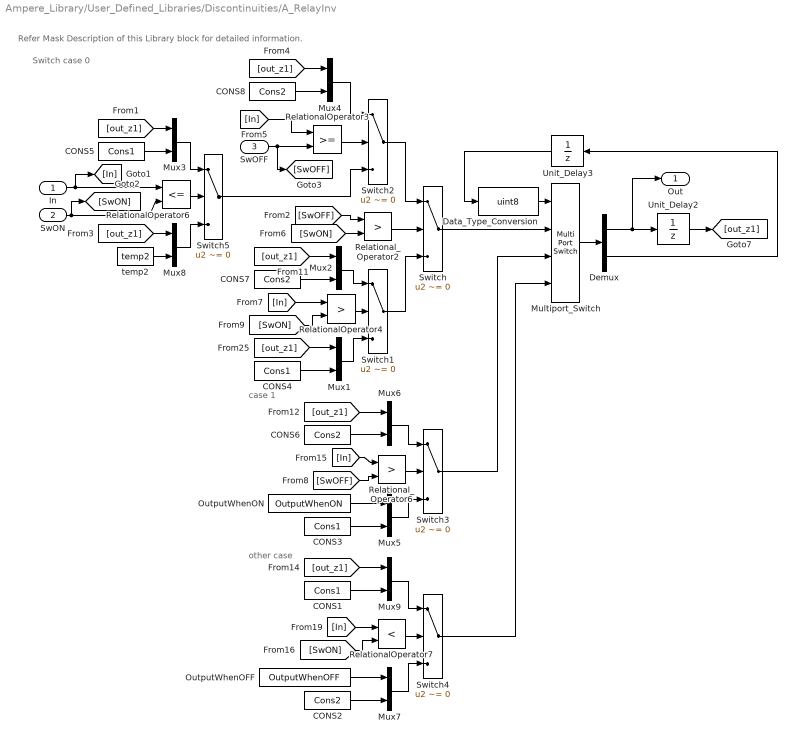
== system Ampere_Library/User_Defined_Libraries/Discontinuities/A_RelayInv ==
  note: Refer Mask Description of this Library block for detailed information.
  note: case 1
  note: Switch case 0
  note: other case
  In : Inport
  SwON : Inport  Port=2
  SwOFF : Inport  Port=3
  CONS{1,3..5} (4 alike) : Constant  Value=Cons1  OutDataTypeStr=Inherit: Inherit via back propagation
  CONS{2,6..8} (4 alike) : Constant  Value=Cons2  OutDataTypeStr=Inherit: Inherit via back propagation
  Data_Type_Conversion : DataTypeConversion  OutDataTypeStr=uint8
      settings: AttributesFormatString=SAT = %<SaturateOnIntegerOverflow>
  Demux : Demux  Outputs=2
  Multiport_Switch : MultiPortSwitch  DataPortOrder=Zero-based contiguous  Inputs=2  DataPortForDefault=Additional data port  DiagnosticForDefault=None  zeroidx=on  RndMeth=Zero  SaturateOnIntegerOverflow=off
      settings: AttributesFormatString=SAT = %<SaturateOnIntegerOverflow>
  Mux{1..9} (9 alike) : Mux  Inputs=2
  OutputWhenOFF : Constant  Value=OutputWhenOFF  OutDataTypeStr=Inherit: Inherit via back propagation
  OutputWhenON : Constant  Value=OutputWhenON  OutDataTypeStr=Inherit: Inherit via back propagation
  RelationalOperator3 : RelationalOperator  OutDataTypeStr=boolean  RndMeth=Zero
  RelationalOperator4 : RelationalOperator  Operator=>  OutDataTypeStr=boolean  RndMeth=Zero
  RelationalOperator6 : RelationalOperator  Operator=<=  OutDataTypeStr=boolean  RndMeth=Zero
  RelationalOperator7 : RelationalOperator  Operator=<  OutDataTypeStr=boolean  RndMeth=Zero
  Relational_Operator2 : RelationalOperator  Operator=>  OutDataTypeStr=boolean  RndMeth=Zero
  Relational_Operator6 : RelationalOperator  Operator=>  OutDataTypeStr=boolean  RndMeth=Zero
  Switch{,1..5} (6 alike) : Switch  Criteria=u2 ~= 0  RndMeth=Zero  SaturateOnIntegerOverflow=off
      settings: AttributesFormatString=SAT = %<SaturateOnIntegerOverflow>
  Unit_Delay2 : UnitDelay  InitialCondition=IniVal  SampleTime=-1  HasFrameUpgradeWarning=on
      settings: AttributesFormatString=Init = %<InitialCondition>\n
  Unit_Delay3 : UnitDelay  InitialCondition=IniVal  SampleTime=-1  HasFrameUpgradeWarning=on
      settings: AttributesFormatString=Init = %<InitialCondition>\n
  temp2 : Constant  Value=temp2  OutDataTypeStr=Inherit: Inherit via back propagation
  Out : Outport
  wires:
  Mux7/1 -> Switch4/3
  [out_z1] -> Mux9/1
  Relational_Operator2/1 -> Switch/2
  CONS2/1 -> Mux7/2
  [In] -> RelationalOperator3/1
  OutputWhenOFF/1 -> Mux7/1
  Mux4/1 -> Switch2/1
  CONS4/1 -> Mux1/2
  [In] -> RelationalOperator7/1
  Unit_Delay3/1 -> Data_Type_Conversion/1
  [SwON] -> RelationalOperator7/2
  OutputWhenON/1 -> Mux5/1
  [In] -> Relational_Operator6/1
  RelationalOperator6/1 -> Switch5/2
  Multiport_Switch/1 -> Demux/1
  [out_z1] -> Mux2/1
  CONS3/1 -> Mux5/2
  Relational_Operator6/1 -> Switch3/2
  Unit_Delay2/1 -> [out_z1]
  Switch/1 -> Multiport_Switch/2
  Mux9/1 -> Switch4/1
  RelationalOperator7/1 -> Switch4/2
  Mux6/1 -> Switch3/1
  [out_z1] -> Mux6/1
  CONS6/1 -> Mux6/2
  RelationalOperator4/1 -> Switch1/2
  [out_z1] -> Mux4/1
  Switch1/1 -> Switch/3
  SwOFF/1 -> RelationalOperator3/2, [SwOFF]
  Mux1/1 -> Switch1/3
  Switch3/1 -> Multiport_Switch/3
  temp2/1 -> Mux8/2
  CONS1/1 -> Mux9/2
  Mux2/1 -> Switch1/1
  Switch2/1 -> Switch/1
  In/1 -> RelationalOperator6/1, [In]
  CONS8/1 -> Mux4/2
  [out_z1] -> Mux8/1
  CONS7/1 -> Mux2/2
  Mux5/1 -> Switch3/3
  Switch4/1 -> Multiport_Switch/4
  CONS5/1 -> Mux3/2
  [out_z1] -> Mux1/1
  Switch5/1 -> Switch2/3
  SwON/1 -> RelationalOperator6/2, [SwON]
  Demux/2 -> Unit_Delay3/1
  Mux8/1 -> Switch5/3
  RelationalOperator3/1 -> Switch2/2
  Mux3/1 -> Switch5/1
  [out_z1] -> Mux3/1
  Data_Type_Conversion/1 -> Multiport_Switch/1
  Demux/1 -> Out/1, Unit_Delay2/1
  [SwON] -> Relational_Operator2/2
  [SwOFF] -> Relational_Operator2/1
  [SwOFF] -> Relational_Operator6/2
  [In] -> RelationalOperator4/1
  [SwON] -> RelationalOperator4/2

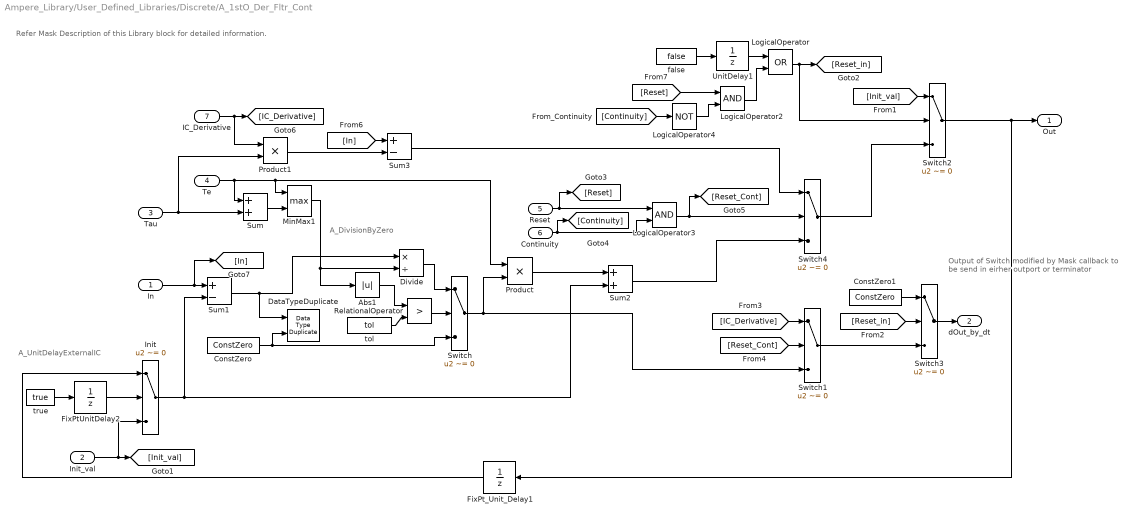
== system Ampere_Library/User_Defined_Libraries/Discrete/A_1stO_Der_Fltr_Cont ==
  note: Output of Switch modified by Mask callback
      | to be send in eirher outport or terminator
  note: A_UnitDelayExternalIC
  note: A_DivisionByZero
  note: Refer Mask Description of this Library block for detailed information.
  In : Inport
  Init_val : Inport  Port=2
  Tau : Inport  Port=3
  Te : Inport  Port=4
  Reset : Inport  Port=5
  Continuity : Inport  Port=6
  IC_Derivative : Inport  Port=7
  Abs1 : Abs  RndMeth=Zero
      settings: AttributesFormatString=SAT = %<SaturateOnIntegerOverflow>
  ConstZero : Constant  Value=ConstZero  OutDataTypeStr=Inherit: Inherit via back propagation
  ConstZero1 : Constant  Value=ConstZero  OutDataTypeStr=Inherit: Inherit via back propagation
  DataTypeDuplicate : DataTypeDuplicate
  Divide : Product  Inputs=*/  RndMeth=Zero  SaturateOnIntegerOverflow=on
      settings: AttributesFormatString=SAT = %<SaturateOnIntegerOverflow>
  FixPtUnitDelay2 : UnitDelay  DisableCoverage=on  InitialCondition=false  SampleTime=-1  HasFrameUpgradeWarning=on
      settings: AttributesFormatString=Init = %<InitialCondition>
  FixPt_Unit_Delay1 : UnitDelay  DisableCoverage=on  InitialCondition=UDEIC_zero  SampleTime=-1  HasFrameUpgradeWarning=on
      settings: AttributesFormatString=Init = %<InitialCondition>
  Init : Switch  Criteria=u2 ~= 0  RndMeth=Zero  ZeroCross=off
      settings: AttributesFormatString=SAT = %<SaturateOnIntegerOverflow>
  LogicalOperator : Logic  Operator=OR  OutDataTypeStr=boolean
  LogicalOperator2 : Logic  OutDataTypeStr=boolean
  LogicalOperator3 : Logic  OutDataTypeStr=boolean
  LogicalOperator4 : Logic  Operator=NOT  OutDataTypeStr=boolean
  MinMax1 : MinMax  Function=max  Inputs=2  InputSameDT=on  RndMeth=Zero
      settings: AttributesFormatString=SAT = %<SaturateOnIntegerOverflow>
  Product : Product  InputSameDT=on  OutDataTypeStr=Inherit: Inherit via back propagation  RndMeth=Zero
      settings: AttributesFormatString=SAT = %<SaturateOnIntegerOverflow>
  Product1 : Product  InputSameDT=on  OutDataTypeStr=Inherit: Inherit via back propagation  RndMeth=Zero
      settings: AttributesFormatString=SAT = %<SaturateOnIntegerOverflow>\n
  RelationalOperator : RelationalOperator  Operator=>  OutDataTypeStr=boolean  RndMeth=Zero
  Sum : Sum  InputSameDT=on  RndMeth=Zero
      settings: AttributesFormatString=SAT = %<SaturateOnIntegerOverflow>
  Sum1 : Sum  Inputs=+-  InputSameDT=on  RndMeth=Zero
      settings: AttributesFormatString=SAT = %<SaturateOnIntegerOverflow>
  Sum2 : Sum  InputSameDT=on  RndMeth=Zero
      settings: AttributesFormatString=SAT = %<SaturateOnIntegerOverflow>
  Sum3 : Sum  Inputs=+-  InputSameDT=on  RndMeth=Zero
      settings: AttributesFormatString=SAT = %<SaturateOnIntegerOverflow>
  Switch : Switch  Criteria=u2 ~= 0  RndMeth=Zero
      settings: AttributesFormatString=SAT = %<SaturateOnIntegerOverflow>
  Switch{1..4} (4 alike) : Switch  Criteria=u2 ~= 0  RndMeth=Zero  SaturateOnIntegerOverflow=off
      settings: AttributesFormatString=SAT = %<SaturateOnIntegerOverflow>
  UnitDelay1 : UnitDelay  InitialCondition=true  SampleTime=-1  HasFrameUpgradeWarning=on
      settings: AttributesFormatString=Init = %<InitialCondition>
  false : Constant  Value=false
  tol : Constant  Value=tol  OutDataTypeStr=Inherit: Inherit via back propagation
  true : Constant  DisableCoverage=on  Value=true
  Out : Outport
  dOut_by_dt : Outport  Port=2
  wires:
  UnitDelay1/1 -> LogicalOperator/1
  Switch/1 -> Switch1/3, Product/2
  Te/1 -> Sum/1, MinMax1/1, Product/1
  IC_Derivative/1 -> [IC_Derivative], Product1/1
  ConstZero1/1 -> Switch3/1
  true/1 -> FixPtUnitDelay2/1
  Divide/1 -> Switch/1
  MinMax1/1 -> Divide/2, Abs1/1
  LogicalOperator/1 -> [Reset_in], Switch2/2
  FixPtUnitDelay2/1 -> Init/2
  Product/1 -> Sum2/1
  LogicalOperator4/1 -> LogicalOperator2/2
  Continuity/1 -> LogicalOperator3/2, [Continuity]
  false/1 -> UnitDelay1/1
  Reset/1 -> [Reset], LogicalOperator3/1
  Sum2/1 -> Switch4/3
  Init/1 -> Sum2/2, Sum1/2
  [IC_Derivative] -> Switch1/1
  Switch3/1 -> dOut_by_dt/1
  Sum3/1 -> Switch4/1
  LogicalOperator3/1 -> [Reset_Cont], Switch4/2
  Switch1/1 -> Switch3/3
  tol/1 -> RelationalOperator/2
  [Reset_in] -> Switch3/2
  LogicalOperator2/1 -> LogicalOperator/2
  [Reset_Cont] -> Switch1/2
  Switch4/1 -> Switch2/3
  [In] -> Sum3/1
  Sum/1 -> MinMax1/2
  Tau/1 -> Product1/2, Sum/2
  [Init_val] -> Switch2/1
  In/1 -> [In], Sum1/1
  ConstZero/1 -> Switch/3, DataTypeDuplicate/2
  Abs1/1 -> RelationalOperator/1
  Init_val/1 -> Init/3, [Init_val]
  [Reset] -> LogicalOperator2/1
  FixPt_Unit_Delay1/1 -> Init/1
  Sum1/1 -> Divide/1, DataTypeDuplicate/1
  Switch2/1 -> Out/1, FixPt_Unit_Delay1/1
  [Continuity] -> LogicalOperator4/1
  RelationalOperator/1 -> Switch/2
  Product1/1 -> Sum3/2
